simulink model "WebcamTester4"  (Simulink 7.3)
settings: Solver=FixedStepDiscrete  StartTime=0.0  StopTime=inf  MaxStep=0.2  RelTol=1e-3
settings Model: Creator=gclayton  LastModifiedBy=wildcat
settings DebuggingCC: InheritedTsInSrcMsg=none
settings RTWCC: SystemTargetFile=rlnx.tlc  GenCodeOnly=on  TemplateMakefile=rlnx_ubuntu.tmf  Description=Linux Real-Time Target  ProcessScript=rlnx_make_rtw_hook
settings RTWCC: CustomInclude=|
  | /usr/local/include/opencv/
  | /usr/local/include/
settings CodeAppCC: GenerateComments=off  SimulinkBlockComments=off
settings STFCustomTargetCC: ModelReferenceCompliant=off  MatFileLogging=on  SystemTargetFile=rlnx.tlc
settings GRTTargetCC: ModelReferenceCompliant=off  ParMdlRefBuildCompliant=off  CompOptLevelCompliant=off
settings CustomProperty: DataType=string  Value=-lm -ldl /usr/local/lib/libopencv_highgui.so.2.4
settings EnumStrPairs: String=PC

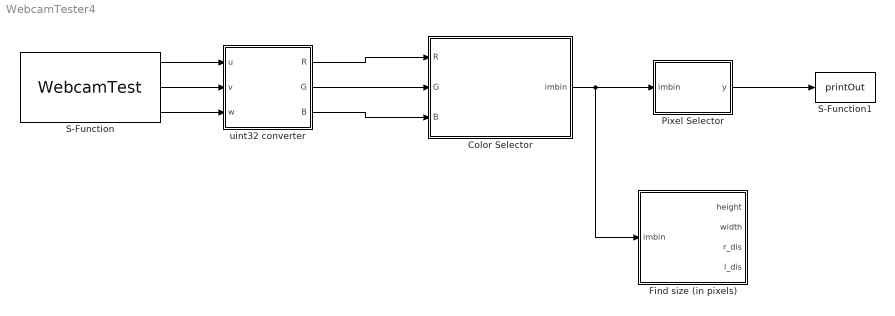
== system WebcamTester4 ==
  Color Selector : Stateflow chart  TreatAsAtomicUnit=on
  Find size (in pixels) : Stateflow chart  TreatAsAtomicUnit=on
  Pixel Selector : Stateflow chart
  S-Function : S-Function  FunctionName=WebcamTest  EnableBusSupport=off
  S-Function1 : S-Function  FunctionName=printOut  EnableBusSupport=off
  uint32 converter : Stateflow chart
  wires:
  S-Function/1 -> uint32 converter/1(u)
  S-Function/2 -> uint32 converter/2(v)
  S-Function/3 -> uint32 converter/3(w)
  uint32 converter/2(G) -> Color Selector/2(G)
  uint32 converter/3(B) -> Color Selector/3(B)
  Color Selector/1(imbin) -> Pixel Selector/1(imbin), Find size (in pixels)/1(imbin)
  uint32 converter/1(R) -> Color Selector/1(R)
  Pixel Selector/1(y) -> S-Function1/1

== matlab function uint32 converter ==
  data: u input double; R output double; v input double; w input double; G output double; B output double
function [R,G,B]= fcn(u,v,w)

R = uint32(u);
G = uint32(v);
B = uint32(w);

== matlab function Pixel Selector ==
  data: imbin input double; y output double
function y = fcn(imbin)
%#eml

imsize = size(imbin);
red_pix = 0;

for (imh = 1:imsize(1,1));
    for (iml = 1:imsize(1,2));
        im_pix = imbin(imh,iml);     
        if (im_pix == 1)
           red_pix = red_pix+1;
        end
    end
end

y = uint32(red_pix);

== matlab function Color Selector ==
  data: R input double; G input double; B input double; imbin output double
function imbin  = color_selection(R,G,B)

imsize = size(R);
imsize = size(G);
imsize = size(B);

R1 = zeros(imsize);
G1 = zeros(imsize);
B1 = zeros(imsize);
imbin = zeros(imsize);

for (imh = 1:imsize(1,1));
    for (iml = 1:imsize(1,2));
        imR = R(imh,iml);
        imG = G(imh,iml);
        imB = B(imh,iml);
        if (imR >= 170) && (imR <= 255) && (imG >= 15) && (imG <= 70) && (imB >= 70) && (imB <= 130)
            R1(imh,iml) = 255;
            G1(imh,iml) = 255;
            B1(imh,iml) = 255;
            imbin(imh,iml) = 1;
        end
    end
end

== matlab function Find size (in pixels) ==
  data: imbin input double; height output double; width output double; r_dis output double; l_dis output double
function [height,width,r_dis,l_dis] = hw_find(imbin)

imsize=size(imbin);

height = 0;
width = 0;
height_sum = 0;
width_sum = 0;
marker = 0;
obstart = 0;

for (imh = 1:imsize(1,1));
    width_sum = 0;
    for (iml = 1:imsize(1,2));
        imloc = imbin(imh,iml);
        if (imloc == 1)
            width_sum=width_sum+1;
        end
    end
    if (width_sum >= 6)
        height = height+1;
    end
end



for (iml = 1:imsize(1,2));
    height_sum = 0;
    for (imh = 1:imsize(1,1));
        imloc = imbin(imh,iml);
        if (imloc == 1)
            height_sum=height_sum+1;
        end
    end
    if (height_sum >= 6)
        width = width+1;
        if (marker == 0)
            marker = 1;
            obstart = iml;
        end
    end
end

obend = obstart + width;

r_dis = obstart;
l_dis = imsize(1,2) - obend;
